simulink model "zynqRadioQPSKTransmitRepeatRecordSL"  (R2016a)
settings: Solver=FixedStepDiscrete  SolverMode=SingleTasking  StartTime=0.0  StopTime=sdrqpsktx.FrameTime*199  RelTol=1e-3
PreLoadFcn:
  | sdrqpsktx = zynqRadioQPSKTxAD9361AD9364SL_init;
InitFcn:
  | sdrqpsktx =  zynqRadioQPSKTxAD9361AD9364SL_init;
StopFcn:
  | save('zynqRadioQPSKTransmitData.mat','zynqRadioQPSKTransmitData');
undefined symbols (not defined in the file or in its folder): gcbh, rcfiltgaincompat
libraries: commrandsrc3 x1, dspsigops x1, commsequence2 x1, sdrzblksprivate x1, commdigbbndpm3 x1, commfilt2 x1
CloseFcn:
  | clear sdrqpsktx genMsg;
Description:
  | Implement a QPSK Transmitter prototype using SDR hardware
settings Model: FPTRunName=Active  ModifiedByFormat=The MathWorks Inc.  Creator=The MathWorks, Inc.  LastModifiedBy=The MathWorks Inc.
settings DataIOCC: LimitDataPoints=on  SaveFormat=Array  SaveOutput=off  SaveTime=off
settings OptimizationCC: BooleanDataType=off  DefaultParameterBehavior=Inlined  ExpressionDepthLimit=2147483647  LocalBlockOutputs=off
settings DebuggingCC: AlgebraicLoopMsg=error  UnderspecifiedInitializationDetection=Classic  MergeDetectMultiDrivingBlocksExec=none  SolverPrmCheckMsg=warning  SingleTaskRateTransMsg=error  FcnCallInpInsideContextMsg=UseLocalSettings  AllowSymbolicDim=off  StateNameClashWarn=warning
settings HardwareCC: ProdBitPerPointer=32  ProdLargestAtomicFloat=None  ProdIntDivRoundTo=Undefined  ProdEndianess=Unspecified  ProdWordSize=32  ProdHWDeviceType=32-bit Generic  TargetBitPerPointer=64  TargetLongLongMode=on  TargetIntDivRoundTo=Zero  TargetEndianess=LittleEndian  TargetWordSize=64  TargetHWDeviceType=Generic->MATLAB Host Computer  ProdEqTarget=off
settings ModelReferenceCC: PropagateSignalLabelsOutOfModel=off
settings RTWCC: CustomSourceCode=|
  | #include <stdio.h>
  | #include <stdlib.h>
settings GRTTargetCC: CombineOutputUpdateFcns=off  GRTInterface=on
settings ConfigComp: CovModelRefEnable=Off  CovSFcnEnable=off

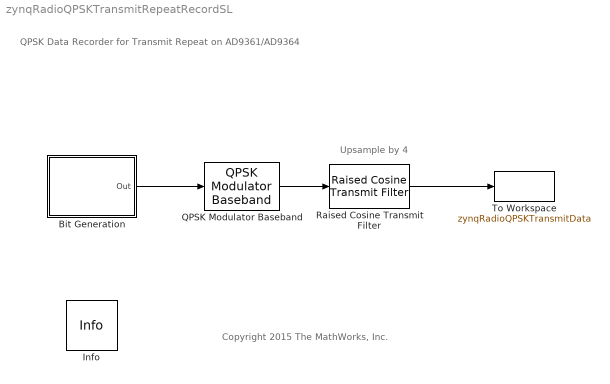
== system zynqRadioQPSKTransmitRepeatRecordSL ==
  note: Upsample by 4
  note: QPSK Data Recorder for Transmit Repeat on AD9361/AD9364
  note: Copyright 2015 The MathWorks, Inc.
  Bit Generation : Subsystem
      mask Display: disp('Bits Generation')
  Info : sdrzblksprivate/Info  SystemSampleTime=-1
  QPSK Modulator Baseband : commdigbbndpm3/QPSK Modulator Baseband  InType=Bit  Enc=Gray  Ph=pi/4  outDtype=double  outWordLen=16  outUDDataType=sfix(16)  outFracLenMode=Best precision  outFracLen=15  outDataTypeStr=double  outLastDataTypeStr=double
  Raised Cosine Transmit Filter : commfilt2/Raised Cosine Transmit Filter  filtType=Square root  R=0.5  filtSpan=2*((sdrqpsktx.RCFiltSpan)/2)  N=sdrqpsktx.Upsampling  filterGain=rcfiltgaincompat(gcbh)  InputProcessing=Columns as channels (frame based)  RateOptions=Enforce single-rate processing  framing=Mute  checkCoeff=off  variableName=rcTxFilt1  checkGain=Normalized  sampMode=Mute  saveAsFlag=0  currentFiltSpan=2*((sdrqpsktx.RCFiltSpan)/2)  D=(sdrqpsktx.RCFiltSpan)/2  launchFVT=off  roundingMode=Floor  overflowMode=off  coeffDataTypeStr=Inherit: Same word length as input  coeffMin=[]  coeffMax=[]  coeffLastDataTypeStr=Inherit: Same word length as input  outputDataTypeStr=Inherit: Same as accumulator  outputMin=[]  outputMax=[]  outputLastDataTypeStr=Inherit: Same as accumulator
  To Workspace : ToWorkspace  VariableName=zynqRadioQPSKTransmitData  SampleTime=-1
      settings: MaxDataPoints=40000  Save2DSignal=2-D array (concatenate along first dimension)
  wires:
  QPSK Modulator Baseband/1 -> Raised Cosine Transmit Filter/1
  Bit Generation/1(Out) -> QPSK Modulator Baseband/1
  Raised Cosine Transmit Filter/1 -> To Workspace/1

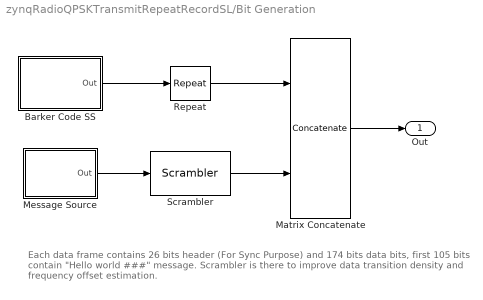
== system zynqRadioQPSKTransmitRepeatRecordSL/Bit Generation ==
  note: Each data frame contains 26 bits header (For Sync Purpose) and 174 bits data bits,
      | first 105 bits contain "Hello world ###" message. Scrambler is there to improve data
      | transition density and frequency offset estimation.
  Barker Code SS : Subsystem
      mask Display: disp('Unipolar\nBarker Code')
  Matrix Concatenate : Concatenate  Mode=Multidimensional array
  Message Source : Subsystem
      mask Display: disp('Message\nSource')
  Repeat : dspsigops/Repeat  N=2  InputProcessing=Columns as channels (frame based)  RateOptions=Enforce single-rate processing  ic=0  mode=Unused parameter value
  Scrambler : commsequence2/Scrambler  M=2  poly=[1 1 1 0 1]  iniStaSource=Dialog Parameter  ini_sta=[0 0 0 0]  resetViaPort=off
  Out : Outport
  wires:
  Barker Code SS/1(Out) -> Repeat/1
  Matrix Concatenate/1 -> Out/1
  Message Source/1(Out) -> Scrambler/1
  Repeat/1 -> Matrix Concatenate/1
  Scrambler/1 -> Matrix Concatenate/2

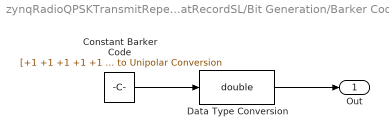
== system zynqRadioQPSKTransmitRepeatRecordSL/Bit Generation/Barker Code SS ==
  Constant Barker Code : Constant  Value=|  VectorParams1D=off
      | [+1 +1 +1 +1 +1 -1 -1 +1 +1 -1 +1 -1 +1
      | ].' > 0  % Bipolar to Unipolar Conversion
  Data Type Conversion : DataTypeConversion  OutDataTypeStr=double
  Out : Outport
  wires:
  Constant Barker Code/1 -> Data Type Conversion/1
  Data Type Conversion/1 -> Out/1

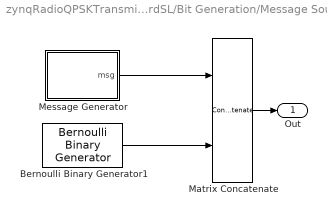
== system zynqRadioQPSKTransmitRepeatRecordSL/Bit Generation/Message Source ==
  Bernoulli Binary Generator1 : commrandsrc3/Bernoulli Binary Generator  ProbabilityOfZero=0.5  SeedSource=Parameter  Seed=61  SampleTime=sdrqpsktx.FrameTime/(sdrqpsktx.DataLength-sdrqpsktx.MsgLength)  SamplesPerFrame=sdrqpsktx.DataLength-sdrqpsktx.MsgLength  OutputDataType=double  SimulateUsing=Interpreted execution
  Matrix Concatenate : Concatenate  Mode=Multidimensional array
  Message Generator : MATLAB Function  TreatAsAtomicUnit=on
  Out : Outport
  wires:
  Message Generator/1(msg) -> Matrix Concatenate/1
  Bernoulli Binary Generator1/1 -> Matrix Concatenate/2
  Matrix Concatenate/1 -> Out/1

== matlab function zynqRadioQPSKTransmitRepeatRecordSL/Bit Generation/Message Source/Message Generator ==
  data: msg output size=[sdrqpsktx.MsgLength, 1]
function msg = genMsg
%#codegen
persistent msgStrSet count;
if isempty(msgStrSet)
    count = 0;
    msgStrSet = ['Hello world 000';...
              'Hello world 001';...
              'Hello world 002';...
              'Hello world 003';...
              'Hello world 004';...
              'Hello world 005';...
              'Hello world 006';...
              'Hello world 007';...
              'Hello world 008';...
              'Hello world 009';...
              'Hello world 010';...
              'Hello world 011';...
              'Hello world 012';...
              'Hello world 013';...
              'Hello world 014';...
              'Hello world 015';...
              'Hello world 016';...
              'Hello world 017';...
              'Hello world 018';...
              'Hello world 019';...
              'Hello world 020';...
              'Hello world 021';...
              'Hello world 022';...
              'Hello world 023';...
              'Hello world 024';...
              'Hello world 025';...
              'Hello world 026';...
              'Hello world 027';...
              'Hello world 028';...
              'Hello world 029';...
              'Hello world 030';...
              'Hello world 031';...
              'Hello world 032';...
              'Hello world 033';...
              'Hello world 034';...
              'Hello world 035';...
              'Hello world 036';...
              'Hello world 037';...
              'Hello world 038';...
              'Hello world 039';...
              'Hello world 040';...
              'Hello world 041';...
              'Hello world 042';...
              'Hello world 043';...
              'Hello world 044';...
              'Hello world 045';...
              'Hello world 046';...
              'Hello world 047';...
              'Hello world 048';...
              'Hello world 049';...
              'Hello world 050';...
              'Hello world 051';...
              'Hello world 052';...
              'Hello world 053';...
              'Hello world 054';...
              'Hello world 055';...
              'Hello world 056';...
              'Hello world 057';...
              'Hello world 058';...
              'Hello world 059';...
              'Hello world 060';...
              'Hello world 061';...
              'Hello world 062';...
              'Hello world 063';...
              'Hello world 064';...
              'Hello world 065';...
              'Hello world 066';...
              'Hello world 067';...
              'Hello world 068';...
              'Hello world 069';...
              'Hello world 070';...
              'Hello world 071';...
              'Hello world 072';...
              'Hello world 073';...
              'Hello world 074';...
              'Hello world 075';...
              'Hello world 076';...
              'Hello world 077';...
              'Hello world 078';...
              'Hello world 079';...
              'Hello world 080';...
              'Hello world 081';...
              'Hello world 082';...
              'Hello world 083';...
              'Hello world 084';...
              'Hello world 085';...
              'Hello world 086';...
              'Hello world 087';...
              'Hello world 088';...
              'Hello world 089';...
              'Hello world 090';...
              'Hello world 091';...
              'Hello world 092';...
              'Hello world 093';...
              'Hello world 094';...
              'Hello world 095';...
              'Hello world 096';...
              'Hello world 097';...
              'Hello world 098';...
              'Hello world 099'];              
end
msgStr = msgStrSet(count+1,:);
msgBin = de2bi(int8(msgStr),7,'left-msb');
msg = reshape(double(msgBin).',105,1);
count = mod(count+1,100);
